simulink model "Main_simulation_gio"  (R2021b)
settings: Solver=FixedStepAuto  StartTime=0.0  StopTime=Time  FixedStep=0.1  RelTol=1e-13  AbsTol=1e-19
values from neighbouring files (symbols this model uses):
  a = 8.6251e06    (= 8625100)    [main_code.m]
  A_BN_0 = eye(3)    [main_code.m]
  A_rw = [1 0 0 1/sqrt(3);         0 1 0 1/sqrt(3) ... (first row only)    [main_code.m]
  A_rw_star = [5/6 -1/6 -1/6;              -1/6  5/6 -1/6 ... (first row only)    [main_code.m]
  c = 2.99792*10^8    (= 299792000)    [main_code.m]
  e = 0.1195    [main_code.m]
  G = [gn, gm, gvali, gsvi]    [main_code.m]
  H = [hn, hm, hvali, hsvi]    [main_code.m]
  i = 0.3815    [main_code.m]
  MB = [1; 0.3; 0.3; 0.3]    [main_code.m]
  mr = 1.2*1e-4    (= 0.00012)    [main_code.m]
  mu_P = G * Mt    (= 398527110340000)    [main_code.m]
  omega_0 = [w_0x; w_0y; w_0z]    [main_code.m]
  p_acc = 0.5    [main_code.m]
  rho_d_MB = 0.1    [main_code.m]
  rho_d_SP = 0.1    [main_code.m]
  rho_s_MB = 0.5    [main_code.m]
  rho_s_SP = 0.1    [main_code.m]
  sig_b = sig_b^2    [main_code.m]
  sig_n = 0.15*pi/180/3600/sqrt(t_sample)    [main_code.m]
  SP = [3; 0.3; 1; 0.1]    [main_code.m]
  T = 2*pi / n    [main_code.m]
  t_sample = 1    [main_code.m]
  theta_0 = 0    [main_code.m]
undefined symbols (not defined in the file or in its folder): magnitude, theta0
libraries: matrix_library x13, vrlib x7, simulink x3, simulink_extras x1
(part 1 of 5)
settings Model: SimulationMode=accelerator  Creator=adity  LastModifiedBy=adity
settings SolverCC: ZeroCrossControl=DisableAll

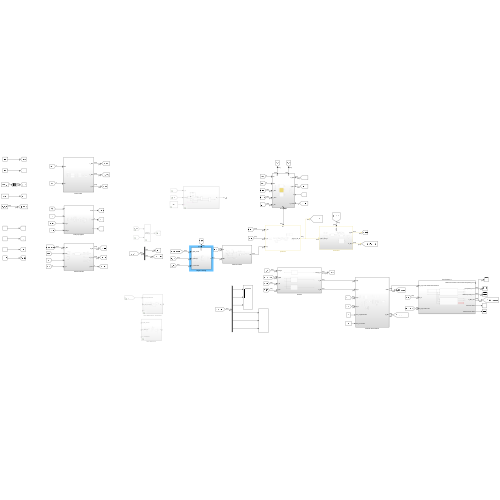
[thumbnail: Simulink's stored preview of the top-level diagram]
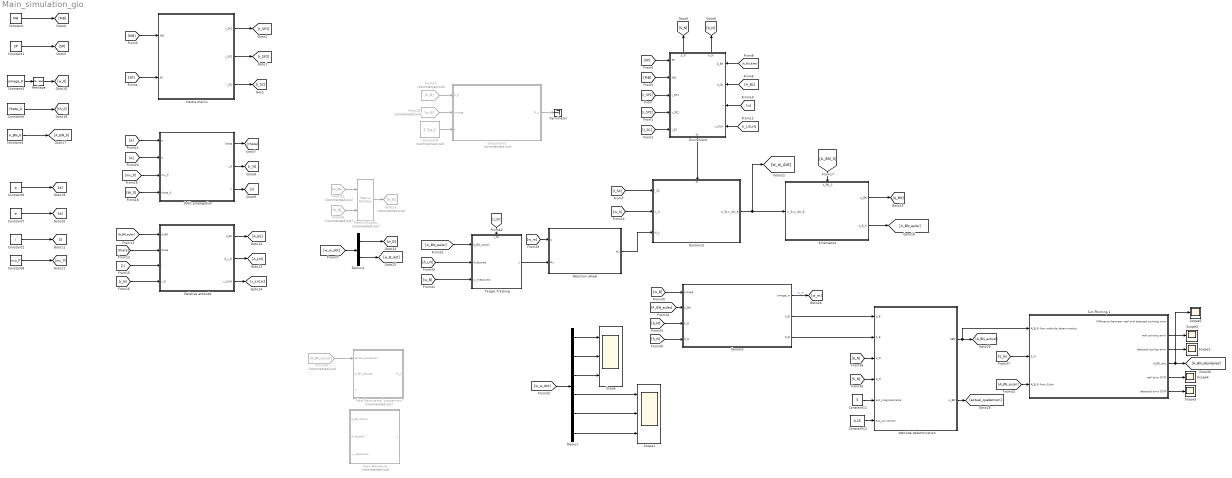
== system Main_simulation_gio ==
  Attitude determination : Subsystem
  Constant : Constant  Value=MB
  Constant1 : Constant  Value=SP
  Constant11 : Constant  Value=5
  Constant12 : Constant  Value=0.25
  Constant2 : Constant  Value=i
  Constant3 : Constant  Value=omega_0
  Constant4 : Constant  Value=A_BN_0
  Constant5 : Constant  Value=theta_0
  Constant6 : Constant  Value=a
  Constant7 : Constant  Value=e
  Constant8 : Constant  Value=mu_P
  Constant9 : Constant  Commented=on  Value=3.5e-2
  Demux : Demux  Outputs=6
  Demux1 : Demux  Outputs=2
  Dynamics : Subsystem
      settings: PortSchema="{\"entries\":[{\"content\":{\"sides\":[{\"content\":{\"connectorIds\":[\"In1\",\"In2\",\"In3\"]},\"type\":\"ConnectorPlacement.EquallySpacedRectSide\",\"uuid\":\"0fb0fd28-732a-45b7-951f-4b0b2306202c\"},{\"content\":{\"connectorIds\":[\"Out1\"],\"side\":\"RIGHT\"},\"type\":\"ConnectorPlacement.EquallySpacedRectSide\",\"uuid\":\"160a6d95-5e8b-4088-9ac4-372e2ef53b1e\"},{\"content\":{\"connectorIds\":[\"In4\"],\"side\":\"TOP\"},\"type\":\"ConnectorPlacement.EquallySpacedRectSide\",\"uuid\":\"bc0d773d-9b3c-40c2-804a-fc9efd6e220c\"}]},\"type\":\"ConnectorPlacement.EquallySpacedConnector\",\"uuid\":\"1f85a25c-c8d4-4d9d-9994-483d99135538\"}],\"packageUris\":[\"http://schema.mathworks.com/mf0/Connector/R2020b\"],\"version\":\"1.0\"}"
  Enviroment : Subsystem
      settings: PortSchema="{\"entries\":[{\"content\":{\"sides\":[{\"content\":{\"connectorIds\":[\"Out2\",\"Out3\"]},\"type\":\"ConnectorPlacement.EquallySpacedRectSide\",\"uuid\":\"77a65197-c5ef-4c05-af97-bd670bb59a1b\"},{\"content\":{\"connectorIds\":[\"Out1\"],\"side\":\"RIGHT\"},\"type\":\"ConnectorPlacement.EquallySpacedRectSide\",\"uuid\":\"f4905732-994b-44e8-915f-1f1165b6d340\"},{\"content\":{\"connectorIds\":[\"In1\",\"In2\",\"In3\",\"In4\",\"In5\"],\"side\":\"TOP\"},\"type\":\"ConnectorPlacement.EquallySpacedRectSide\",\"uuid\":\"dbb628bc-072b-4daa-a580-a056bf799753\"},{\"content\":{\"connectorIds\":[\"In6\",\"In7\",\"In8\",\"In9\"],\"side\":\"BOTTOM\"},\"type\":\"ConnectorPlacement.EquallySpacedRectSide\",\"uuid\":\"e6af6235-b92e-4098-9bbc-91b77f168ead\"}]},\"type\":\"ConnectorPlacement.EquallySpacedConnector\",\"uuid\":\"a4645f0d-8f51-4ba7-9ec5-d423e83ccc17\"}],\"packageUris\":[\"http://schema.mathworks.com/mf0/Connector/R2020b\"],\"version\":\"1.0\"}"
  From22 : From  Commented=on  GotoTag=A_BN
  From23 : From  Commented=on  GotoTag=b_B
  From26 : From  Commented=on  GotoTag=b_N
  From28 : From  Commented=on  GotoTag=w_B
  From38 : From  Commented=on  GotoTag=A_BN_actual
  Goto23 : Goto  Commented=on  GotoTag=b_B
  Inertia matrix : Subsystem
  Kinematics : Subsystem
      settings: PortSchema="{\"entries\":[{\"content\":{\"sides\":[{\"content\":{\"connectorIds\":[\"In1\"]},\"type\":\"ConnectorPlacement.EquallySpacedRectSide\",\"uuid\":\"b4580536-f47d-4a76-9d7a-ad9e45e6fd22\"},{\"content\":{\"connectorIds\":[\"Out1\",\"Out2\"],\"side\":\"RIGHT\"},\"type\":\"ConnectorPlacement.EquallySpacedRectSide\",\"uuid\":\"4273ed6e-d469-4a82-9e71-da4fb1c9f709\"},{\"content\":{\"connectorIds\":[\"In2\"],\"side\":\"TOP\"},\"type\":\"ConnectorPlacement.EquallySpacedRectSide\",\"uuid\":\"bac57a2b-a638-4d55-8f6f-550bb52319aa\"}]},\"type\":\"ConnectorPlacement.EquallySpacedConnector\",\"uuid\":\"29527554-7b77-4957-9d93-347c44cffae5\"}],\"packageUris\":[\"http://schema.mathworks.com/mf0/Connector/R2020b\"],\"version\":\"1.0\"}"
  Matrix Multiply : Product  Commented=on  Multiplication=Matrix(*)
  Orbit propagation : Subsystem
  Reaction wheel : Subsystem
  Relative attitude : Subsystem
  Reshape : Reshape  OutputDimensionality=Column vector (2-D)
  Scope : Scope  NumInputPorts=3
  Scope1 : Scope  NumInputPorts=3
  Scope{2..6} (5 alike) : Scope
  Sensors : Subsystem
  Slew Manoevre : Subsystem  Commented=on
  "Slew Manouevre \"quaternion\"" : Subsystem  Commented=on
  Subsystem1 : Subsystem  Commented=on
  Sun Pointing 1 : Subsystem
  Target Tracking : Subsystem
      settings: PortSchema="{\"entries\":[{\"content\":{\"sides\":[{\"content\":{\"connectorIds\":[\"In1\",\"In2\",\"In3\"]},\"type\":\"ConnectorPlacement.EquallySpacedRectSide\",\"uuid\":\"1538af5c-7ca3-4c69-907f-3af05bd2e46a\"},{\"content\":{\"connectorIds\":[\"Out1\"],\"side\":\"RIGHT\"},\"type\":\"ConnectorPlacement.EquallySpacedRectSide\",\"uuid\":\"fe4d23c6-7042-48db-bda4-c7db1868d73a\"},{\"content\":{\"connectorIds\":[\"In4\"],\"side\":\"TOP\"},\"type\":\"ConnectorPlacement.EquallySpacedRectSide\",\"uuid\":\"8091eb5d-cc3c-4ce8-99cb-f347939312a6\"}]},\"type\":\"ConnectorPlacement.EquallySpacedConnector\",\"uuid\":\"01b1afd0-a44e-4fda-a912-00799ef3cdac\"}],\"packageUris\":[\"http://schema.mathworks.com/mf0/Connector/R2020b\"],\"version\":\"1.0\"}"
  Terminator : Terminator
  wires:
  Inertia matrix/3(I_SC) -> [I_SC]
  Inertia matrix/2(r_SP2) -> [r_SP2]
  Inertia matrix/1(r_SP1) -> [r_SP1]
  [r_SP1] -> Enviroment/3(r_SP1)
  [r_SP2] -> Enviroment/4(r_SP2)
  [I_SC] -> Enviroment/5(I_SC)
  Constant/1 -> [MB]
  Constant1/1 -> [SP]
  [MB] -> Inertia matrix/1(MB)
  [SP] -> Inertia matrix/2(SP)
  [MB] -> Enviroment/2(MB)
  [SP] -> Enviroment/1(SP)
  Enviroment/1(M) -> Dynamics/4(M)
  [I_SC] -> Dynamics/1(I_SC)
  Enviroment/2(S_N) -> [S_N]
  Enviroment/3(b_N) -> [b_N]
  [A_BN_euler] -> Enviroment/6(A_BN)
  [A_BL] -> Enviroment/7(A_BL)
  [n] -> Enviroment/8(n)
  [r_LVLH] -> Enviroment/9(r_LVLH)
  Orbit propagation/1(theta) -> [theta]
  Orbit propagation/2(r_N) -> [r_N]
  Orbit propagation/3(n) -> [n]
  [theta] -> Relative attitude/2(theta)
  [A_BN_euler] -> Relative attitude/1(A_BN)
  [w_0] -> Dynamics/2(w_0)
  Constant2/1 -> [i]
  [i] -> Relative attitude/3(i)
  Relative attitude/1(A_BL) -> [A_BL]
  Relative attitude/2(A_L_N) -> [A_LN]
  Dynamics/1(w_B,w_dot_B) -> [w_w_dot], Kinematics/1(w_B,w_dot_B)
  [r_N] -> Relative attitude/4(r_N)
  Relative attitude/3(r_LVLH) -> [r_LVLH]
  Kinematics/1(q_BN) -> [q_BN]
  Kinematics/2(A_B_N) -> [A_BN_euler]
  [A_BN_0] -> Kinematics/2(A_BN_0)
  Constant4/1 -> [A_BN_0]
  Constant5/1 -> [th_0]
  [th_0] -> Orbit propagation/4(theta_0)
  Constant6/1 -> [a]
  Constant7/1 -> [e]
  Constant8/1 -> [mu_P]
  [mu_P] -> Orbit propagation/3(mu_P)
  [e] -> Orbit propagation/2(e)
  [a] -> Orbit propagation/1(a)
  Demux/1 -> Scope/1
  Demux/2 -> Scope/2
  Demux/3 -> Scope/3
  Demux/4 -> Scope1/1
  Demux/5 -> Scope1/2
  Demux/6 -> Scope1/3
  [w_w_dot] -> Demux/1
  From22/1 -> Matrix Multiply/1
  From26/1 -> Matrix Multiply/2
  Matrix Multiply/1 -> Goto23/1
  From23/1 -> Subsystem1/1(b_b)
  [w_w_dot] -> Demux1/1
  Demux1/1 -> [w_B]
  Demux1/2 -> [w_B_dot]
  Constant9/1 -> Subsystem1/3(K)
  From28/1 -> Subsystem1/2(omega)
  Constant3/1 -> Reshape/1
  Reshape/1 -> [w_0]
  Target Tracking/1(u) -> Reaction wheel/2(Mc)
  Reaction wheel/1(Mr) -> Dynamics/3(M_c)
  From38/1 -> "Slew Manouevre \"quaternion\""/1(actual quaternion)
  [w_m] -> Reaction wheel/1(w)
  [A_LN] -> Target Tracking/2(A_desired)
  [w_B] -> Target Tracking/3(w_measured)
  Subsystem1/1(M_c) -> Terminator/1
  [w_B] -> Sensors/1(omega)
  [A_BN_euler] -> Sensors/2(A_BN)
  [b_N] -> Sensors/3(b_N)
  [S_N] -> Sensors/4(S_N)
  Sensors/1(omega_m) -> [w_m]  "w_m"
  Sensors/2(b_B) -> Attitude determination/1(b_B)
  Sensors/3(S_B) -> Attitude determination/2(S_B)
  Constant12/1 -> Attitude determination/6(acc_sun sensor)
  Constant11/1 -> Attitude determination/5(acc_magnetometre)
  [S_N] -> Attitude determination/4(S_N)
  [b_N] -> Attitude determination/3(b_N)
  Sun Pointing 1/4(A_BN_des) -> Scope6/1, [A_BN_desidered]
  [S_N] -> Sun Pointing 1/2(S_N)
  [A_BN_euler] -> Sun Pointing 1/3(A_B_N from Euler)
  Attitude determination/1(ABN) -> Sun Pointing 1/1(A_B_N from attitude determination), [A_BN_actual]
  Sun Pointing 1/3(detected pointig error) -> Scope2/1
  Sun Pointing 1/2(real pointing error) -> Scope3/1
  Sun Pointing 1/5(real error DCM) -> Scope4/1
  Sun Pointing 1/6(detected error DCM) -> Scope5/1
  Attitude determination/2(q_BN) -> [actual_quaternion]
  [A_BN_euler] -> Target Tracking/1(A_BN_actual)
  [I_SC] -> Target Tracking/4(I_SC)

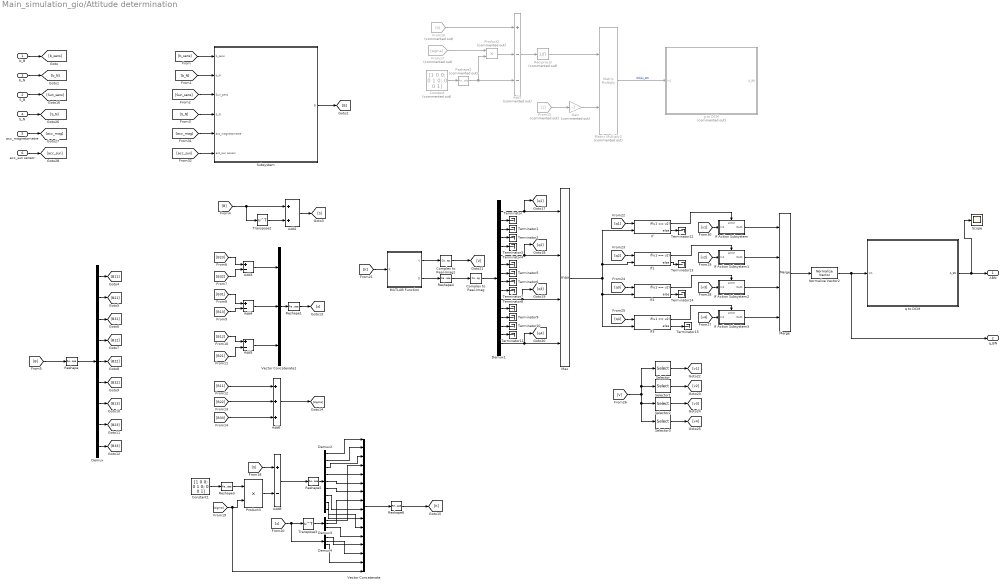
== system Main_simulation_gio/Attitude determination ==
  b_B : Inport
  S_B : Inport  Port=2
  b_N : Inport  Port=3
  S_N : Inport  Port=4
  acc_magnetometre : Inport  Port=5
  acc_sun sensor : Inport  Port=6
  Add2 : Sum
  Add{3..5,8} (4 alike) : Sum  Inputs=+-
  Add6 : Sum  Inputs=+++
  Add7 : Sum  Commented=on  Inputs=+--
  Complex to Real-Imag : ComplexToRealImag  Output=Real
  Complex to Real-Imag1 : ComplexToRealImag  Output=Real
  Constant : Constant  Commented=on  Value=[1 0 0; 0 1 0; 0 0 1]  VectorParams1D=off
  Constant1 : Constant  Value=[1 0 0; 0 1 0; 0 0 1]  VectorParams1D=off
  Demux : Demux  Outputs=9
  Demux1 : Demux  Outputs=16
  Demux2 : Demux  Outputs=9
  Demux3 : Demux  Outputs=3
  Demux4 : Demux  Outputs=3
  From15 : From  Commented=on  GotoTag=z
  From16 : From  Commented=on  GotoTag=S
  From17 : From  Commented=on  GotoTag=sigma
  Gain : Gain  Commented=on  Gain=-1
  If{,1..3} (4 alike) : If  NumInputs=2  IfExpression=u1 == u2
  If Action Subsystem : Subsystem  TreatAsAtomicUnit=on
  If Action Subsystem1 : Subsystem  TreatAsAtomicUnit=on
  If Action Subsystem2 : Subsystem  TreatAsAtomicUnit=on
  If Action Subsystem3 : Subsystem  TreatAsAtomicUnit=on
  MATLAB Function : MATLAB Function  TreatAsAtomicUnit=on
  Matrix Multiply2 : Product  Commented=on  Multiplication=Matrix(*)
  Max : MinMax  Function=max  Inputs=4
  Merge : Merge  Inputs=4
  Normalize Vector2 : vrlib/Utilities/Normalize Vector  maxzero=0
  Product2 : Product  Commented=on
  Product3 : Product
  Reciprocal : Product  Commented=on  Inputs=/
  Reshape{,1,4..5} (4 alike) : Reshape  OutputDimensionality=Column vector (2-D)
  Reshape2 : Reshape  Commented=on  OutputDimensionality=Customize  OutputDimensions=[3,3]
  Reshape3 : Reshape  OutputDimensionality=Customize  OutputDimensions=[3,3]
  Reshape6 : Reshape  OutputDimensionality=Customize  OutputDimensions=[4,4]
  Scope : Scope
  Selector : Selector  NumberOfDimensions=2  InputPortWidth=3  IndexOptions=Index vector (dialog),Index vector (dialog)  Indices=[1 2 3 4],1  OutputSizes=1,1
  Selector1 : Selector  NumberOfDimensions=2  InputPortWidth=3  IndexOptions=Index vector (dialog),Index vector (dialog)  Indices=[1 2 3 4],2  OutputSizes=1,1
  Selector2 : Selector  NumberOfDimensions=2  InputPortWidth=3  IndexOptions=Index vector (dialog),Index vector (dialog)  Indices=[1 2 3 4],3  OutputSizes=1,1
  Selector3 : Selector  NumberOfDimensions=2  InputPortWidth=3  IndexOptions=Index vector (dialog),Index vector (dialog)  Indices=[1 2 3 4],4  OutputSizes=1,1
  Subsystem : Subsystem
  Terminator{,1..15} (16 alike) : Terminator
  Transpose2 : Math  Operator=transpose  SaturateOnIntegerOverflow=on
  Transpose3 : Math  Operator=transpose  SaturateOnIntegerOverflow=on
  Vector Concatenate : Concatenate  NumInputs=16
  Vector Concatenate1 : Concatenate  NumInputs=3
  g to DCM : Subsystem  Commented=on
  q to DCM : Subsystem
  ABN : Outport
  q_BN : Outport  Port=2
  wires:
  [B] -> Transpose2/1, Add2/1
  Transpose2/1 -> Add2/2
  Add2/1 -> [S]
  [B] -> Reshape/1
  Reshape/1 -> Demux/1
  Demux/1 -> [B11]
  Demux/2 -> [B21]
  Demux/3 -> [B31]
  Demux/4 -> [B12]
  Demux/5 -> [B22]
  Demux/6 -> [B32]
  Demux/7 -> [B13]
  Demux/8 -> [B23]
  Demux/9 -> [B33]
  [B23] -> Add3/1
  [B32] -> Add3/2
  [B31] -> Add4/1
  [B13] -> Add4/2
  [B12] -> Add5/1
  [B21] -> Add5/2
  Add3/1 -> Vector Concatenate1/1
  Add4/1 -> Vector Concatenate1/2
  Add5/1 -> Vector Concatenate1/3
  Vector Concatenate1/1 -> Reshape1/1
  Reshape1/1 -> [z]
  [B11] -> Add6/1
  [B22] -> Add6/2
  [B33] -> Add6/3
  Add6/1 -> [sigma]
  From15/1 -> Gain/1
  Constant/1 -> Reshape2/1
  From17/1 -> Product2/1
  Reshape2/1 -> Add7/3, Product2/2
  From16/1 -> Add7/1
  Product2/1 -> Add7/2
  Add7/1 -> Reciprocal/1
  Reciprocal/1 -> Matrix Multiply2/1
  Gain/1 -> Matrix Multiply2/2
  Matrix Multiply2/1 -> g to DCM/1(In1)  "Gibbs_BN"
  Constant1/1 -> Reshape3/1
  Reshape3/1 -> Product3/1
  [sigma] -> Vector Concatenate/16, Product3/2
  Product3/1 -> Add8/2
  [S] -> Add8/1
  Add8/1 -> Reshape5/1
  MATLAB Function/2(D) -> Reshape4/1
  Demux1/2 -> Terminator/1
  Demux1/3 -> Terminator1/1
  Demux1/4 -> Terminator2/1
  Demux1/5 -> Terminator3/1
  Demux1/6 -> [q2], Max/2
  Demux1/7 -> Terminator4/1
  Demux1/8 -> Terminator5/1
  Demux1/9 -> Terminator6/1
  Demux1/10 -> Terminator7/1
  Demux1/11 -> [q3], Max/3
  Demux1/16 -> [q4], Max/4
  Demux1/12 -> Terminator8/1
  Demux1/13 -> Terminator9/1
  Demux1/14 -> Terminator10/1
  Demux1/15 -> Terminator11/1
  Reshape4/1 -> Complex to Real-Imag/1
  Max/1 -> If3/2, If2/2, If1/2, If/2
  Demux1/1 -> [q1], Max/1
  [q1] -> If/1
  [q2] -> If1/1
  [q4] -> If3/1
  [q3] -> If2/1
  MATLAB Function/1(V) -> Complex to Real-Imag1/1
  Selector1/1 -> [v2]
  Selector3/1 -> [v4]
  Selector2/1 -> [v3]
  Selector/1 -> [v1]
  [V] -> Selector/1, Selector1/1, Selector3/1, Selector2/1
  If/1 -> If Action Subsystem/Action
  If/2 -> Terminator12/1
  If1/2 -> Terminator13/1
  If2/2 -> Terminator14/1
  If3/2 -> Terminator15/1
  If Action Subsystem/1(Out1) -> Merge/1
  If1/1 -> If Action Subsystem1/Action
  If2/1 -> If Action Subsystem2/Action
  If3/1 -> If Action Subsystem3/Action
  If Action Subsystem3/1(Out1) -> Merge/4
  If Action Subsystem2/1(Out1) -> Merge/3
  If Action Subsystem1/1(Out1) -> Merge/2
  [v4] -> If Action Subsystem3/1(In1)
  [v1] -> If Action Subsystem/1(In1)
  [v2] -> If Action Subsystem1/1(In1)
  [v3] -> If Action Subsystem2/1(In1)
  q to DCM/1(A_BN) -> Scope/1, ABN/1
  Merge/1 -> Normalize Vector2/1
  Reshape5/1 -> Demux2/1
  Demux2/1 -> Vector Concatenate/1
  Demux2/2 -> Vector Concatenate/2
  Demux2/3 -> Vector Concatenate/3
  [z] -> Demux4/1, Transpose3/1
  Transpose3/1 -> Demux3/1
  Demux3/1 -> Vector Concatenate/4
  Demux2/4 -> Vector Concatenate/5
  Demux2/5 -> Vector Concatenate/6
  Demux2/6 -> Vector Concatenate/7
  Demux3/2 -> Vector Concatenate/8
  Demux2/7 -> Vector Concatenate/9
  Demux2/8 -> Vector Concatenate/10
  Demux2/9 -> Vector Concatenate/11
  Demux3/3 -> Vector Concatenate/12
  Demux4/2 -> Vector Concatenate/14
  Demux4/1 -> Vector Concatenate/13
  Demux4/3 -> Vector Concatenate/15
  Vector Concatenate/1 -> Reshape6/1
  Reshape6/1 -> [K]
  Complex to Real-Imag/1 -> Demux1/1
  Normalize Vector2/1 -> q_BN/1, q to DCM/1(In1)
  Complex to Real-Imag1/1 -> [V]
  [K] -> MATLAB Function/1(K)
  Subsystem/1(B) -> [B]
  b_B/1 -> [b_sens]
  b_N/1 -> [b_N]
  S_B/1 -> [Sun_sens]
  S_N/1 -> [S_N]
  acc_magnetometre/1 -> [acc_mag]
  acc_sun sensor/1 -> [acc_sun]
  [b_sens] -> Subsystem/1(b_sens)
  [b_N] -> Subsystem/2(b_N)
  [Sun_sens] -> Subsystem/3(Sun_sens)
  [S_N] -> Subsystem/4(S_N)
  [acc_mag] -> Subsystem/5(acc_magnetometre)
  [acc_sun] -> Subsystem/6(acc_sun sensor)

== system Main_simulation_gio/Dynamics ==
  I_SC : Inport
  w_0 : Inport  Port=2
  M_c : Inport  Port=3
  M : Inport  Port=4
  Add : Sum
  Cross Product : vrlib/Utilities/Cross Product
  Demux : Demux  Outputs=3
  Gain5 : Gain  Gain=-1
  Integrator4 : Integrator  InitialConditionSource=external  InitialCondition=omega_0
  Mux : Mux  Inputs=2
  Product6 : Product  Multiplication=Matrix(*)
  Product7 : Product  Multiplication=Matrix(*)
  Reciprocal : Product  Inputs=/  Multiplication=Matrix(*)
  Scope : Scope  NumInputPorts=3
  Scope1 : Scope
  Sum2 : Sum
  w_B,w_dot_B : Outport
  wires:
  Sum2/1 -> Product7/2
  Product6/1 -> Cross Product/2
  Product7/1 -> [w_dot_B], Integrator4/1
  Cross Product/1 -> Gain5/1
  Gain5/1 -> Sum2/1
  Integrator4/1 -> [w_B], Demux/1, Cross Product/1, Product6/2
  I_SC/1 -> [I_SC]
  [I_SC] -> Product6/1
  [I_SC] -> Reciprocal/1
  Reciprocal/1 -> Product7/1
  w_0/1 -> [w_0]
  [w_0] -> Integrator4/2
  Demux/2 -> Scope/2  "om_y"
  Demux/1 -> Scope/1  "om_x"
  Demux/3 -> Scope/3  "om_z"
  Add/1 -> Sum2/2
  M_c/1 -> Add/2
  Mux/1 -> w_B,w_dot_B/1
  [w_B] -> Mux/1
  [w_dot_B] -> Mux/2
  M/1 -> Add/1, Scope1/1

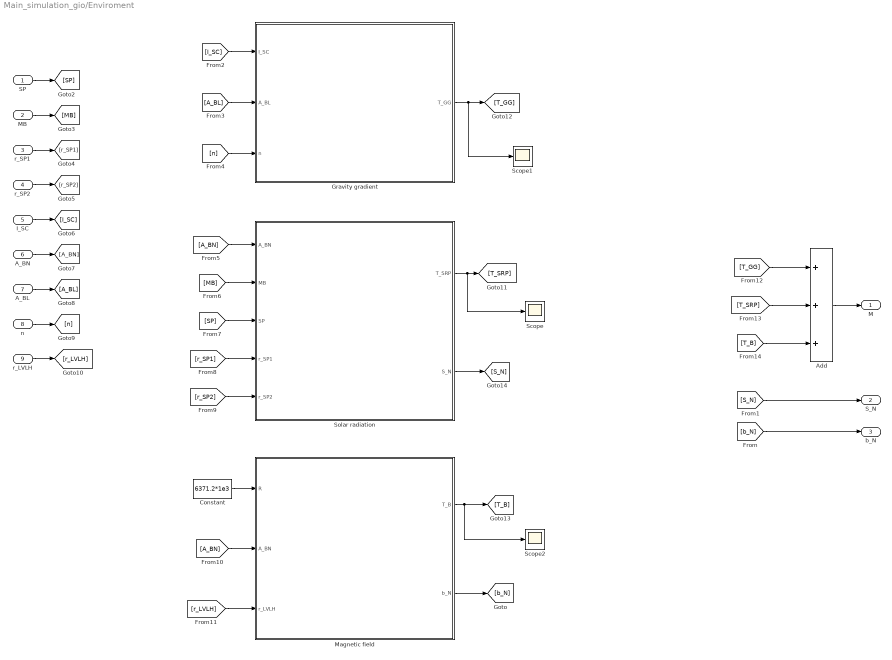
== system Main_simulation_gio/Enviroment ==
  SP : Inport
  MB : Inport  Port=2
  r_SP1 : Inport  Port=3
  r_SP2 : Inport  Port=4
  I_SC : Inport  Port=5
  A_BN : Inport  Port=6
  A_BL : Inport  Port=7
  n : Inport  Port=8
  r_LVLH : Inport  Port=9
  Add : Sum  Inputs=+++
  Constant : Constant  Value=6371.2*1e3
  Gravity gradient : Subsystem
  Magnetic field : Subsystem
  Scope : Scope
  Scope1 : Scope
  Scope2 : Scope
  Solar radiation : Subsystem
  M : Outport
  S_N : Outport  Port=2
  b_N : Outport  Port=3
  wires:
  Add/1 -> M/1
  Constant/1 -> Magnetic field/1(R)
  [b_N] -> b_N/1
  [S_N] -> S_N/1
  SP/1 -> [SP]
  MB/1 -> [MB]
  r_SP1/1 -> [r_SP1]
  r_SP2/1 -> [r_SP2]
  I_SC/1 -> [I_SC]
  A_BN/1 -> [A_BN]
  A_BL/1 -> [A_BL]
  n/1 -> [n]
  r_LVLH/1 -> [r_LVLH]
  Magnetic field/2(b_N) -> [b_N]
  Solar radiation/1(T_SRP) -> Scope/1, [T_SRP]
  Gravity gradient/1(T_GG) -> Scope1/1, [T_GG]
  Magnetic field/1(T_B) -> Scope2/1, [T_B]
  [I_SC] -> Gravity gradient/1(I_SC)
  [A_BL] -> Gravity gradient/2(A_BL)
  [n] -> Gravity gradient/3(n)
  [A_BN] -> Solar radiation/1(A_BN)
  [MB] -> Solar radiation/2(MB)
  [SP] -> Solar radiation/3(SP)
  [r_SP1] -> Solar radiation/4(r_SP1)
  [r_SP2] -> Solar radiation/5(r_SP2)
  [A_BN] -> Magnetic field/2(A_BN)
  [r_LVLH] -> Magnetic field/3(r_LVLH)
  Solar radiation/2(S_N) -> [S_N]
  [T_GG] -> Add/1
  [T_SRP] -> Add/2
  [T_B] -> Add/3

== system Main_simulation_gio/Inertia matrix ==
  note: I_SP is for 2 solar panels
  note: a lato corto, b lato lungo h spessore
      | lato lungo asse x solar panel
      | lato corto asse z solar panel
      | lato lungo asse y main body
      | lato corto asse x main body
      | spessore asse z main body
  MB : Inport
  SP : Inport  Port=2
  Complex to Real-Imag : ComplexToRealImag  Output=Real
  Constant : Constant  Value=[19.5 0 0; 0 19 0; 0 0 12.6]  VectorParams1D=off
  Demux : Demux
  Demux1 : Demux
  MATLAB Function : MATLAB Function  TreatAsAtomicUnit=on
  Main body : Subsystem
  Reshape : Reshape  OutputDimensionality=Customize  OutputDimensions=[3,3]
  Solar panel : Subsystem
  Sum : Sum
  Terminator : Terminator
  Terminator1 : Terminator
  Transport theorem : Subsystem
  r_SP : Subsystem
  r_SP1 : Outport
  r_SP2 : Outport  Port=2
  I_SC : Outport  Port=3
  wires:
  MB/1 -> Demux1/1
  Demux/1 -> [m_SP]
  Transport theorem/1(I_SP_B) -> Sum/1
  [r_SP1] -> Transport theorem/2(r_SP)
  Main body/1(I_MB) -> Sum/2
  [m_SP] -> Transport theorem/3(m_SP)
  r_SP/1(r_SP1) -> [r_SP1]
  [r_SP1] -> r_SP1/1
  [r_SP2] -> r_SP2/1
  r_SP/2(r_SP2) -> [r_SP2]
  Demux/2 -> [a_SP]
  Demux/3 -> [b_SP]
  Demux/4 -> [h_SP]
  [a_SP] -> Solar panel/2(a_SP)
  [b_SP] -> Solar panel/3(b_SP)
  [m_SP] -> Solar panel/1(m_SP)
  [h_SP] -> Solar panel/4(h_SP)
  [b_SP] -> r_SP/1(b_SP)
  Demux1/4 -> [h_MB]
  Demux1/3 -> [b_MB]
  Demux1/2 -> [a_MB]
  Demux1/1 -> [m_MB]
  [m_MB] -> Main body/1(m_MB)
  [a_MB] -> Main body/2(a_MB)
  [b_MB] -> Main body/3(b_MB)
  [h_MB] -> Main body/4(h_MB)
  [a_MB] -> r_SP/2(a_MB)
  Solar panel/1(I_SP) -> [I_SP]
  SP/1 -> Demux/1
  [I_SC] -> I_SC/1
  [I_SP] -> Transport theorem/1(I_SP)
  Sum/1 -> MATLAB Function/1(u)
  MATLAB Function/1(V) -> Terminator/1
  MATLAB Function/2(D) -> Complex to Real-Imag/1
  Complex to Real-Imag/1 -> Terminator1/1
  Constant/1 -> Reshape/1
  Reshape/1 -> [I_SC]

== system Main_simulation_gio/Kinematics ==
  w_B,w_dot_B : Inport
  A_BN_0 : Inport  Port=2
  DCM to quaternion : Subsystem
  Demux : Demux  Outputs=2
  Gain : Gain  Gain=1/2
  Integrator : Integrator  InitialConditionSource=external  InitialCondition=[0; 0; 0; 1]
  Matrix Multiply : Product  Multiplication=Matrix(*)
  Normalisation : Subsystem
  Reshape : Reshape  OutputDimensionality=Column vector (2-D)
  Subsystem : Subsystem
  Terminator : Terminator
  q to DCM : Subsystem
  q_BN : Outport
  A_B_N : Outport  Port=2
  wires:
  w_B,w_dot_B/1 -> Demux/1
  Demux/1 -> [w_B]
  Demux/2 -> Terminator/1
  A_BN_0/1 -> [A_BN_0]
  [q_0] -> Integrator/2
  [w_B] -> Subsystem/1(w_B)
  DCM to quaternion/1(q) -> [q_0]
  Subsystem/1(OMEGA) -> [OMEGA]
  Reshape/1 -> Normalisation/1(In1)
  Integrator/1 -> Reshape/1  "q(t)"
  [OMEGA] -> Gain/1
  Gain/1 -> Matrix Multiply/1
  Normalisation/1(Out1) -> Matrix Multiply/2, [q_BN]  "q(t)"
  Matrix Multiply/1 -> Integrator/1  "dq/dt"
  [A_BN_0] -> DCM to quaternion/1(DCM)
  [q_BN] -> q_BN/1
  [A_BN] -> A_B_N/1
  q to DCM/1(A_BN) -> [A_BN]
  [q_BN] -> q to DCM/1(q_BN)

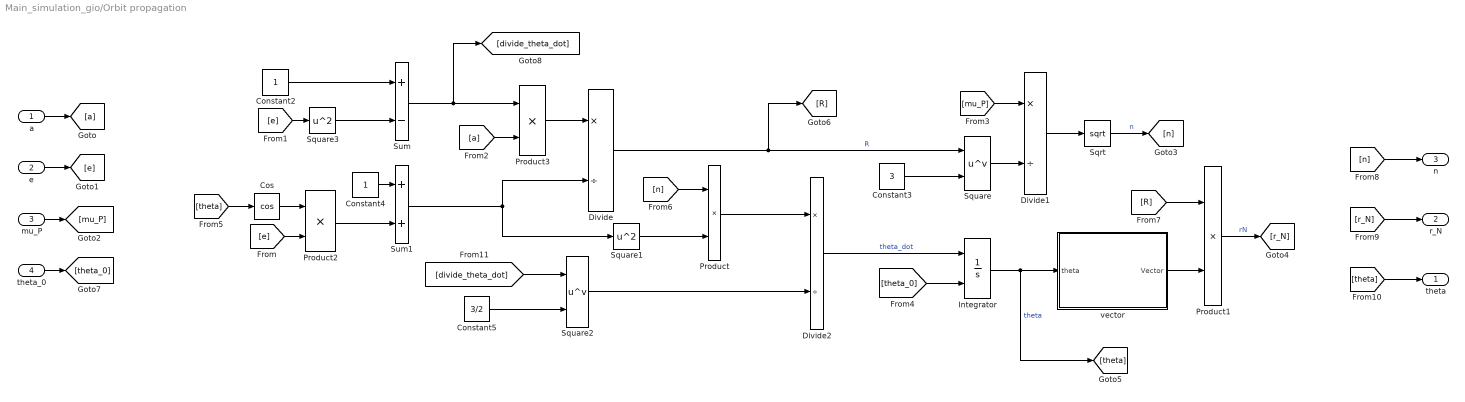
== system Main_simulation_gio/Orbit propagation ==
  a : Inport
  e : Inport  Port=2
  mu_P : Inport  Port=3
  theta_0 : Inport  Port=4
  Constant2 : Constant
  Constant3 : Constant  Value=3
  Constant4 : Constant
  Constant5 : Constant  Value=3/2
  Cos : Trigonometry  Operator=cos
  Divide : Product  Inputs=*/
  Divide1 : Product  Inputs=*/
  Divide2 : Product  Inputs=*/
  Integrator : Integrator  InitialConditionSource=external  InitialCondition=theta0
  Product{,1..3} (4 alike) : Product
  Sqrt : Sqrt  SaturateOnIntegerOverflow=on
  Square : Math  Operator=pow  SaturateOnIntegerOverflow=on
  Square1 : Math  Operator=square  SaturateOnIntegerOverflow=on
  Square2 : Math  Operator=pow  SaturateOnIntegerOverflow=on
  Square3 : Math  Operator=square  SaturateOnIntegerOverflow=on
  Sum : Sum  Inputs=+-
  Sum1 : Sum
  vector : Subsystem
  theta : Outport
  r_N : Outport  Port=2
  n : Outport  Port=3
  wires:
  Constant2/1 -> Sum/1
  Square3/1 -> Sum/2
  Sum/1 -> [divide_theta_dot], Product3/1
  Product3/1 -> Divide/1
  Constant4/1 -> Sum1/1
  Sum1/1 -> Square1/1, Divide/2
  Product2/1 -> Sum1/2
  Cos/1 -> Product2/1
  Integrator/1 -> [theta], vector/1(theta)  "theta"
  Divide1/1 -> Sqrt/1
  [mu_P] -> Divide1/1
  Square/1 -> Divide1/2
  Divide/1 -> [R], Square/1  "R"
  Constant3/1 -> Square/2
  Sqrt/1 -> [n]  "n"
  Square1/1 -> Product/2
  Constant5/1 -> Square2/2
  Product/1 -> Divide2/1
  Divide2/1 -> Integrator/1  "theta_dot"
  vector/1(Vector) -> Product1/2
  Square2/1 -> Divide2/2
  a/1 -> [a]
  e/1 -> [e]
  mu_P/1 -> [mu_P]
  [e] -> Product2/2
  [e] -> Square3/1
  [a] -> Product3/2
  [theta_0] -> Integrator/2
  Product1/1 -> [r_N]  "rN"
  [theta] -> Cos/1
  [n] -> Product/1
  [R] -> Product1/1
  [n] -> n/1
  [r_N] -> r_N/1
  [theta] -> theta/1
  theta_0/1 -> [theta_0]
  [divide_theta_dot] -> Square2/1

== system Main_simulation_gio/Reaction wheel ==
  w : Inport
  Mc : Inport  Port=2
  A : Constant  Value=A_rw
  A_star : Constant  Value=A_rw_star
  Add : Sum  Inputs=--
  Constant : Constant  Value=[0 0 0 0]
  Cross Product : matrix_library/Cross Product
      settings: SourceProductBaseCode=SL
  Cross Product1 : matrix_library/Cross Product
      settings: SourceProductBaseCode=SL
  Gain : Gain  Gain=-1
  Integrator : Integrator  InitialConditionSource=external
  Matrix Multiply{,1..3} (4 alike) : Product  Multiplication=Matrix(*)
  Reshape : Reshape  OutputDimensionality=Column vector (2-D)
  Reshape1 : Reshape  OutputDimensionality=Column vector (2-D)
  Sum : Sum  Inputs=|++
  Mr : Outport
  wires:
  Integrator/1 -> [h_r], Matrix Multiply/2
  A/1 -> [A_rw], Matrix Multiply/1
  w/1 -> [omega], Cross Product/1
  Matrix Multiply/1 -> Cross Product/2
  Cross Product/1 -> Sum/1
  Mc/1 -> Reshape1/1
  Sum/1 -> Matrix Multiply1/2
  A_star/1 -> Gain/1
  Gain/1 -> Matrix Multiply1/1
  Matrix Multiply1/1 -> Integrator/1, Matrix Multiply2/2
  Constant/1 -> Reshape/1
  Reshape/1 -> Integrator/2
  Reshape1/1 -> Sum/2
  [A_rw] -> Matrix Multiply2/1
  Matrix Multiply2/1 -> Add/1
  Add/1 -> Mr/1
  [omega] -> Cross Product1/1
  Matrix Multiply3/1 -> Cross Product1/2
  [A_rw] -> Matrix Multiply3/1
  [h_r] -> Matrix Multiply3/2
  Cross Product1/1 -> Add/2

== system Main_simulation_gio/Relative attitude ==
  A_BN : Inport
  theta : Inport  Port=2
  i : Inport  Port=3
  r_N : Inport  Port=4
  A_LN : Subsystem
  MatrixMultiply : Product  Multiplication=Matrix(*)
  MatrixMultiply1 : Product  Multiplication=Matrix(*)
  Transpose : Math  Operator=transpose  SaturateOnIntegerOverflow=on
  A_BL : Outport
  A_L_N : Outport  Port=2
  r_LVLH : Outport  Port=3
  wires:
  Transpose/1 -> MatrixMultiply/2
  MatrixMultiply/1 -> A_BL/1  "A_BL"
  theta/1 -> [theta]
  A_BN/1 -> [A_BN]
  [theta] -> A_LN/1(theta)
  A_LN/1(A_L_N) -> [A_LN]
  [i] -> A_LN/2(i)
  i/1 -> [i]
  [A_BN] -> MatrixMultiply/1
  [A_LN] -> Transpose/1
  [A_LN] -> A_L_N/1
  MatrixMultiply1/1 -> r_LVLH/1  "A_BL"
  [A_LN] -> MatrixMultiply1/1
  r_N/1 -> [r_N]
  [r_N] -> MatrixMultiply1/2

== system Main_simulation_gio/Sensors ==
  omega : Inport
  A_BN : Inport  Port=2
  b_N : Inport  Port=3
  S_N : Inport  Port=4
  Gyroscopes : Subsystem
  Magnetometer1 : Subsystem
  Sun sensor : Subsystem
  omega_m : Outport
  b_B : Outport  Port=2
  S_B : Outport  Port=3
  wires:
  omega/1 -> Gyroscopes/1(omega)
  Gyroscopes/1(omega_m) -> omega_m/1
  b_N/1 -> Magnetometer1/2(b_N)
  Magnetometer1/1(b_B) -> b_B/1
  Sun sensor/1(S_B) -> S_B/1
  A_BN/1 -> Sun sensor/2(A_BN), Magnetometer1/1(A_BN)
  S_N/1 -> Sun sensor/1(S_N)

== system Main_simulation_gio/Slew Manoevre ==
  A_BN_actual : Inport
  A_desired : Inport  Port=2
  w_measured : Inport  Port=3
  Demux : Demux  Outputs=3
  Gain : Gain  Gain=-1
  Gain1 : Gain  Gain=-1
  Matrix Multiply : Product  Multiplication=Matrix(*)
  Mux : Mux  Inputs=3
  Product : Product
  Product1 : Product
  Reshape : Reshape  OutputDimensionality=Customize  OutputDimensions=[3,1]
  Reshape1 : Reshape  OutputDimensionality=Column vector (2-D)
  Reshape2 : Reshape  OutputDimensionality=Column vector (2-D)
  Scope{,1..3} (4 alike) : Scope
  Selector : Selector  NumberOfDimensions=2  InputPortWidth=3  IndexOptions=Index vector (dialog),Index vector (dialog)  Indices=2,1  OutputSizes=1,1
  Selector1 : Selector  NumberOfDimensions=2  InputPortWidth=3  IndexOptions=Index vector (dialog),Index vector (dialog)  Indices=3,1  OutputSizes=1,1
  Selector2 : Selector  NumberOfDimensions=2  InputPortWidth=3  IndexOptions=Index vector (dialog),Index vector (dialog)  Indices=3,2  OutputSizes=1,1
  Sum : Sum  Inputs=|+|-|
  Sum1 : Sum  Inputs=|+|+|
  Terminator : Terminator
  Terminator1 : Terminator
  To Workspace : ToWorkspace  VariableName=error  SaveFormat=Timeseries  SampleTime=-1
  To Workspace1 : ToWorkspace  VariableName=omega  SaveFormat=Timeseries  SampleTime=-1
  Transpose : Math  Operator=transpose  SaturateOnIntegerOverflow=on
  Transpose1 : Math  Operator=transpose  SaturateOnIntegerOverflow=on
  k1 : Constant  Value=9.99e-2
  k2 : Constant  Value=1.25e-3
  u : Outport
  wires:
  Mux/1 -> Reshape/1, Demux/1, Scope/1
  w_measured/1 -> To Workspace1/1, Scope3/1, Product/1
  Demux/3 -> Terminator1/1
  Demux/2 -> Terminator/1
  Demux/1 -> To Workspace/1
  Gain1/1 -> Product/2
  k1/1 -> Gain1/1
  Gain/1 -> Product1/2
  k2/1 -> Gain/1
  Product/1 -> Reshape1/1
  Reshape1/1 -> Sum1/2
  Product1/1 -> Reshape2/1
  Transpose/1 -> Matrix Multiply/2
  Selector1/1 -> Mux/2
  Selector/1 -> Mux/1
  Selector2/1 -> Mux/3
  Reshape/1 -> Product1/1
  Sum1/1 -> Scope2/1, u/1
  Reshape2/1 -> Sum1/1
  Sum/1 -> Selector1/1, Selector/1, Selector2/1
  Transpose1/1 -> Sum/1
  Matrix Multiply/1 -> Transpose1/1, Sum/2
  A_BN_actual/1 -> Matrix Multiply/1, Scope1/1
  A_desired/1 -> Transpose/1

== system Main_simulation_gio/Slew Manouevre "quaternion" ==
  actual quaternion : Inport
  A_BN_desired : Inport  Port=2
  ω : Inport  Port=3
  A_B_N to quaternion : Subsystem
  Creation of Q_euler1 : Subsystem
  Demux : Demux
  Gain : Gain  Gain=-1
  Gain2 : Gain  Gain=-2
  Mux : Mux  Inputs=3
  Product : Product  Multiplication=Matrix(*)
  Product1 : Product
  Product2 : Product  Inputs=3
  Reshape : Reshape  OutputDimensionality=Column vector (2-D)
  Scope : Scope
  Scope1 : Scope
  Scope2 : Scope
  Sum : Sum  Inputs=|+|+|
  k1 : Constant  Value=0.5
  k2 : Constant  Value=1e-4
  M_c : Outport
  wires:
  actual quaternion/1 -> Product/2
  Creation of Q_euler1/1(Q_desired) -> Product/1
  A_BN_desired/1 -> A_B_N to quaternion/1(A_B_N from Euler)
  A_B_N to quaternion/1(q_euler) -> Creation of Q_euler1/1(q_desired)
  k1/1 -> Gain/1
  Gain/1 -> Product1/1
  ω/1 -> Scope/1, Product1/2
  [q_error] -> Product2/3
  Product1/1 -> Sum/1
  Product2/1 -> Sum/2
  Product/1 -> Scope1/1, Demux/1
  Demux/1 -> [qe1]
  Demux/4 -> [qe4]
  Demux/3 -> [qe3]
  Demux/2 -> [qe2]
  [qe1] -> Mux/1
  [qe2] -> Mux/2
  [qe3] -> Mux/3
  Mux/1 -> Reshape/1
  Reshape/1 -> Scope2/1, [q_error]
  k2/1 -> Product2/1
  [qe4] -> Gain2/1
  Gain2/1 -> Product2/2
  Sum/1 -> M_c/1

== system Main_simulation_gio/Subsystem1 ==
  b_b : Inport
  omega : Inport  Port=2
  K : Inport  Port=3
  Cross Product : matrix_library/Cross Product
      settings: SourceProductBaseCode=SL
  Cross Product1 : matrix_library/Cross Product
      settings: SourceProductBaseCode=SL
  Divide : Product  Inputs=/*
  Dot Product : DotProduct  InputSameDT=on  OutDataTypeStr=Inherit: Inherit via internal rule
  Gain : Gain  Gain=-1
  Product : Product
  M_c : Outport
  wires:
  b_b/1 -> Cross Product/1, Dot Product/2, Dot Product/1, Cross Product1/2
  omega/1 -> Cross Product/2
  Dot Product/1 -> Divide/1
  Cross Product/1 -> Divide/2
  Divide/1 -> Product/1
  Product/1 -> Cross Product1/1
  Cross Product1/1 -> M_c/1
  K/1 -> Gain/1
  Gain/1 -> Product/2

== system Main_simulation_gio/Sun Pointing 1 ==
  A_B_N from attitude determination : Inport
  S_N : Inport  Port=2
  A_B_N from Euler : Inport  Port=3
  Pointing error with DCM : Subsystem
  Pointing error with quaternions : Subsystem
  Difference between real and detected pointing error : Outport
  real pointing error : Outport  Port=2
  detected pointig error : Outport  Port=3
  A_BN_des : Outport  Port=4
  real error DCM : Outport  Port=5
  detected error DCM : Outport  Port=6
  wires:
  A_B_N from attitude determination/1 -> Pointing error with quaternions/1(A_B_N from attitude determination), Pointing error with DCM/3(A_B_N from attitude determination)
  S_N/1 -> Pointing error with quaternions/2(S_N), Pointing error with DCM/2(S_N)
  A_B_N from Euler/1 -> Pointing error with quaternions/3(A_B_N from Euler), Pointing error with DCM/1(A_B_N from Euler)
  Pointing error with DCM/1(Difference between real and detected pointing error) -> Difference between real and detected pointing error/1
  Pointing error with quaternions/2(detected pointing error) -> detected pointig error/1
  Pointing error with quaternions/1(real pointing error) -> real pointing error/1
  Pointing error with quaternions/3(q_euler) -> ?
  Pointing error with quaternions/4(q_desired) -> ?
  Pointing error with DCM/4(A_BN_des) -> A_BN_des/1
  Pointing error with DCM/2(real error DCM) -> real error DCM/1
  Pointing error with DCM/3(Detected error DCM) -> detected error DCM/1

== system Main_simulation_gio/Target Tracking ==
  A_BN_actual : Inport
  A_desired : Inport  Port=2
  w_measured : Inport  Port=3
  I_SC : Inport  Port=4
  Cross Product : matrix_library/Cross Product
      settings: SourceProductBaseCode=SL
  Demux : Demux  Outputs=3
  Gain : Gain  Gain=-1
  Gain1 : Gain  Gain=-1
  Matrix Multiply : Product  Multiplication=Matrix(*)
  Matrix Multiply1 : Product  Multiplication=Matrix(*)
  Mux : Mux  Inputs=3
  Product : Product
  Product1 : Product
  Reshape : Reshape  OutputDimensionality=Customize  OutputDimensions=[3,1]
  Reshape1 : Reshape  OutputDimensionality=Column vector (2-D)
  Reshape2 : Reshape  OutputDimensionality=Column vector (2-D)
  Scope{,1..4} (5 alike) : Scope
  Selector : Selector  NumberOfDimensions=2  InputPortWidth=3  IndexOptions=Index vector (dialog),Index vector (dialog)  Indices=2,1  OutputSizes=1,1
  Selector1 : Selector  NumberOfDimensions=2  InputPortWidth=3  IndexOptions=Index vector (dialog),Index vector (dialog)  Indices=3,1  OutputSizes=1,1
  Selector2 : Selector  NumberOfDimensions=2  InputPortWidth=3  IndexOptions=Index vector (dialog),Index vector (dialog)  Indices=3,2  OutputSizes=1,1
  Sum : Sum  Inputs=|+|-|
  Sum1 : Sum  Inputs=|+|+|+|
  Terminator : Terminator
  Terminator1 : Terminator
  To Workspace : ToWorkspace  VariableName=error  SaveFormat=Timeseries  SampleTime=-1
  To Workspace1 : ToWorkspace  VariableName=omega  SaveFormat=Timeseries  SampleTime=-1
  Transpose : Math  Operator=transpose  SaturateOnIntegerOverflow=on
  Transpose1 : Math  Operator=transpose  SaturateOnIntegerOverflow=on
  k1 : Constant  Value=9.99e-2
  k2 : Constant  Value=1.5e-3
  u : Outport
  wires:
  A_desired/1 -> Scope4/1, Transpose/1
  A_BN_actual/1 -> Scope1/1, Matrix Multiply/1
  Matrix Multiply/1 -> Sum/2, Transpose1/1
  Transpose1/1 -> Sum/1
  Sum/1 -> Selector2/1, Selector/1, Selector1/1
  Reshape2/1 -> Sum1/1
  Sum1/1 -> u/1, Scope2/1
  Reshape/1 -> Product1/1
  Selector2/1 -> Mux/3
  Selector/1 -> Mux/1
  Selector1/1 -> Mux/2
  Transpose/1 -> Matrix Multiply/2
  Product1/1 -> Reshape2/1
  Reshape1/1 -> Sum1/2
  Product/1 -> Reshape1/1
  k2/1 -> Gain/1
  Gain/1 -> Product1/2
  k1/1 -> Gain1/1
  Gain1/1 -> Product/2
  Demux/1 -> To Workspace/1
  Demux/2 -> Terminator/1
  Demux/3 -> Terminator1/1
  [I_mat] -> Matrix Multiply1/1
  w_measured/1 -> Matrix Multiply1/2, Cross Product/1, Product/1, Scope3/1, To Workspace1/1
  Cross Product/1 -> Sum1/3
  I_SC/1 -> [I_mat]
  Mux/1 -> Scope/1, Demux/1, Reshape/1
  Matrix Multiply1/1 -> Cross Product/2

== system Main_simulation_gio/Attitude determination/If Action Subsystem ==
  In1 : Inport
  Action Port : ActionPort  ActionPortLabel=if(u1 == u2)
  Out1 : Outport
  wires:
  In1/1 -> Out1/1

== system Main_simulation_gio/Attitude determination/If Action Subsystem1 ==
  In1 : Inport
  Action Port : ActionPort  ActionPortLabel=if(u1 == u2)
  Out1 : Outport
  wires:
  In1/1 -> Out1/1

== system Main_simulation_gio/Attitude determination/If Action Subsystem2 ==
  In1 : Inport
  Action Port : ActionPort  ActionPortLabel=if(u1 == u2)
  Out1 : Outport
  wires:
  In1/1 -> Out1/1

== system Main_simulation_gio/Attitude determination/If Action Subsystem3 ==
  In1 : Inport
  Action Port : ActionPort  ActionPortLabel=if(u1 == u2)
  Out1 : Outport
  wires:
  In1/1 -> Out1/1

== system Main_simulation_gio/Attitude determination/Subsystem ==
  b_sens : Inport
  b_N : Inport  Port=2
  Sun_sens : Inport  Port=3
  S_N : Inport  Port=4
  acc_magnetometre : Inport  Port=5
  acc_sun sensor : Inport  Port=6
  Add : Sum
  Add1 : Sum
  Divide : Product  Inputs=*/
  Divide1 : Product  Inputs=*/
  Matrix Multiply : Product  Multiplication=Matrix(*)
  Matrix Multiply1 : Product  Multiplication=Matrix(*)
  Normalize Vector : vrlib/Utilities/Normalize Vector  maxzero=0
  Normalize Vector1 : vrlib/Utilities/Normalize Vector  maxzero=0
  Product : Product
  Product1 : Product
  Transpose : Math  Operator=transpose  SaturateOnIntegerOverflow=on
  Transpose1 : Math  Operator=transpose  SaturateOnIntegerOverflow=on
  B : Outport
  wires:
  Transpose/1 -> Matrix Multiply1/2
  b_N/1 -> Normalize Vector1/1
  S_N/1 -> Transpose1/1
  Divide1/1 -> Product1/2
  Normalize Vector/1 -> Matrix Multiply1/1
  Add/1 -> B/1
  Divide/1 -> Product/2
  Product/1 -> Add/1
  b_sens/1 -> Normalize Vector/1
  Add1/1 -> Divide/2, Divide1/2
  [alpha2] -> Divide1/1
  [alpha1] -> Divide/1
  [alpha1] -> Add1/1
  Transpose1/1 -> Matrix Multiply/2
  acc_sun sensor/1 -> [alpha2]
  Matrix Multiply/1 -> Product1/1
  Matrix Multiply1/1 -> Product/1
  [alpha2] -> Add1/2
  acc_magnetometre/1 -> [alpha1]
  Normalize Vector1/1 -> Transpose/1
  Product1/1 -> Add/2
  Sun_sens/1 -> Matrix Multiply/1

== system Main_simulation_gio/Attitude determination/g to DCM ==
  In1 : Inport
  A_BN : Outport
  wires:
  In1/1 -> A_BN/1

== system Main_simulation_gio/Attitude determination/q to DCM ==
  In1 : Inport
  Add : Sum  Inputs=+-
  Add1 : Sum  Inputs=++-
  Constant : Constant  Value=[1 0 0; 0 1 0; 0 0 1]  VectorParams1D=off
  Demux : Demux
  Gain : Gain  Gain=2
  Gain1 : Gain  Gain=2
  Matrix Multiply : Product  Multiplication=Matrix(*)
  Matrix Multiply2 : Product  Multiplication=Matrix(*)
  Mux : Mux  Inputs=3
  Product : Product
  Product1 : Product
  Product2 : Product
  Reshape : Reshape  OutputDimensionality=Column vector (2-D)
  Reshape1 : Reshape  OutputDimensionality=Customize  OutputDimensions=[3,3]
  Scope : Scope
  Square : Math  Operator=square  SaturateOnIntegerOverflow=on
  Transpose : Math  Operator=transpose  SaturateOnIntegerOverflow=on
  Transpose1 : Math  Operator=transpose  SaturateOnIntegerOverflow=on
  Transpose2 : Math  Operator=transpose  SaturateOnIntegerOverflow=on
  orthonormalization step 1 : Subsystem
  q_cross : Subsystem
  A_BN : Outport
  wires:
  In1/1 -> Demux/1
  Demux/4 -> [q4]
  Demux/1 -> [q1]
  Demux/2 -> [q2]
  Demux/3 -> [q3]
  [q4] -> Square/1
  [q2] -> Mux/2
  [q3] -> Mux/3
  [q1] -> Mux/1
  Mux/1 -> Reshape/1
  Reshape/1 -> [q_vect]
  [q_vect] -> Matrix Multiply/2, Transpose/1
  Transpose/1 -> Matrix Multiply/1
  Matrix Multiply/1 -> Add/2
  Square/1 -> Add/1
  Constant/1 -> Reshape1/1
  Reshape1/1 -> Product1/2
  Product1/1 -> Add1/1
  Matrix Multiply2/1 -> Gain/1
  Gain/1 -> Add1/2
  Transpose1/1 -> Matrix Multiply2/2
  [q_vect] -> Transpose1/1, Matrix Multiply2/1
  Gain1/1 -> Add1/3
  Product/1 -> Gain1/1
  [q4] -> Product/2
  q_cross/1(q_cross) -> Product/1
  Add1/1 -> orthonormalization step 1/1(A*(t))
  [q_vect] -> q_cross/1(q_vect)
  Add/1 -> Product1/1
  Transpose2/1 -> Product2/2
  Product2/1 -> Scope/1
  orthonormalization step 1/1(A_BN*_filtered) -> A_BN/1, Product2/1, Transpose2/1

== system Main_simulation_gio/Enviroment/Gravity gradient ==
  I_SC : Inport
  A_BL : Inport  Port=2
  n : Inport  Port=3
  Constant : Constant  Value=3
  Constant1 : Constant  Value=[1 0 0]
  Demux : Demux  Outputs=9
  Demux1 : Demux  Outputs=3
  Matrix Multiply : Product  Multiplication=Matrix(*)
  Mux : Mux  Inputs=3
  Product{,1..9} (10 alike) : Product
  Reshape : Reshape  OutputDimensionality=Column vector (2-D)
  Reshape1 : Reshape  OutputDimensionality=Column vector (2-D)
  Reshape2 : Reshape  OutputDimensionality=Column vector (2-D)
  Scope : Scope  NumInputPorts=3
  Square : Math  Operator=square  SaturateOnIntegerOverflow=on
  Sum : Sum  Inputs=+-
  Sum1 : Sum  Inputs=+-
  Sum2 : Sum  Inputs=+-
  Terminator{,1..5} (6 alike) : Terminator
  T_GG : Outport
  wires:
  Demux/4 -> Terminator2/1
  Demux1/1 -> Product5/2, Product7/2
  Demux/2 -> Terminator/1
  Product6/1 -> Product9/1
  Sum/1 -> Product1/1
  Product1/1 -> Product6/1
  Demux/7 -> Terminator4/1
  Demux1/3 -> Product6/2, Product8/2
  Demux/1 -> Sum1/1
  Product5/1 -> Product8/1
  Demux/3 -> Terminator1/1
  I_SC/1 -> Reshape1/1
  Matrix Multiply/1 -> Demux1/1
  Demux/9 -> Sum2/2, Sum1/2, Sum/1
  Constant1/1 -> Reshape/1
  Sum1/1 -> Product2/1
  Sum2/1 -> Product3/1
  Product7/1 -> Scope/3, Mux/3
  Mux/1 -> Reshape2/1
  Demux/5 -> Sum/2, Sum2/1
  Demux/8 -> Terminator5/1
  A_BL/1 -> Matrix Multiply/1
  Product4/1 -> Product7/1
  Product8/1 -> Scope/2, Mux/2
  Demux/6 -> Terminator3/1
  Demux1/2 -> Product4/2, Product9/2
  Product2/1 -> Product5/1
  Product9/1 -> Scope/1, Mux/1
  Product3/1 -> Product4/1
  Reshape/1 -> Matrix Multiply/2
  Reshape1/1 -> Demux/1
  Reshape2/1 -> T_GG/1
  Square/1 -> Product/1
  Product/1 -> Product2/2, Product1/2, Product3/2
  Constant/1 -> Product/2
  n/1 -> Square/1

== system Main_simulation_gio/Enviroment/Magnetic field ==
  R : Inport
  A_BN : Inport  Port=2
  r_LVLH : Inport  Port=3
  Cross Product : matrix_library/Cross Product
      settings: SourceProductBaseCode=SL
  b_B : Subsystem
  parasitic torque : Subsystem
  T_B : Outport
  b_N : Outport  Port=2
  wires:
  parasitic torque/1(m_par) -> [m_par]
  b_B/1(b_B) -> [b_B]
  b_B/2(b_N) -> [b_N]
  [m_par] -> Cross Product/1
  [b_B] -> Cross Product/2
  [b_N] -> b_N/1
  A_BN/1 -> [A_BN]
  R/1 -> [R]
  r_LVLH/1 -> [r_LVLH]
  [A_BN] -> b_B/1(A_BN)
  [R] -> b_B/2(R)
  [r_LVLH] -> b_B/3(r_LVLH)
  Cross Product/1 -> T_B/1

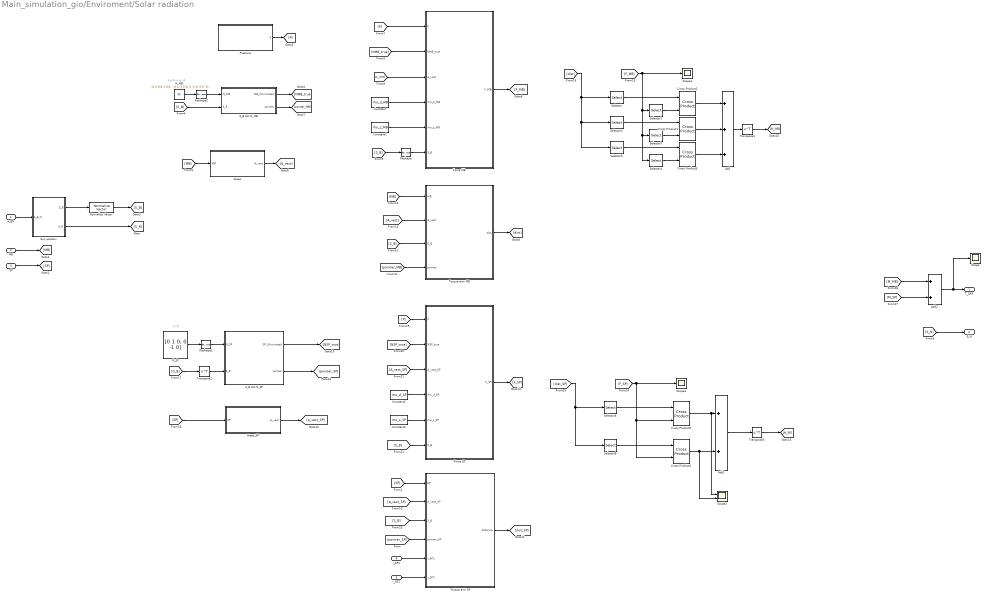
== system Main_simulation_gio/Enviroment/Solar radiation ==
  note: x,y,z,-x,-y,-z
  note: y,-y
  A_BN : Inport
  MB : Inport  Port=2
  SP : Inport  Port=3
  r_SP1 : Inport  Port=4
  r_SP2 : Inport  Port=5
  Add : Sum  Inputs=3
  Add1 : Sum
  Add2 : Sum
  Areas : Subsystem
  Areas_SP : Subsystem
  Constant : Constant  Value=rho_d_MB
  Constant1 : Constant  Value=rho_s_MB
  Constant2 : Constant  Value=rho_d_SP
  Constant3 : Constant  Value=rho_s_SP
  Cross Product{1..5} (5 alike) : matrix_library/Cross Product
      settings: SourceProductBaseCode=SL
  Force MB : Subsystem
  Force SP : Subsystem
  N_MB : Constant  Value=[1 0 0;0 1 0;0 0 1;-1 0 0; 0 -1 0; 0 0 -1]  VectorParams1D=off
  N_SP : Constant  Value=[0 1 0; 0 -1 0]  VectorParams1D=off
  Normalize Vector : vrlib/Utilities/Normalize Vector  maxzero=0
  Pressure : Subsystem
  Reshape : Reshape  OutputDimensionality=Column vector (2-D)
  Reshape1 : Reshape  OutputDimensionality=Customize  OutputDimensions=[2,3]
  Reshape2 : Reshape  OutputDimensionality=Customize  OutputDimensions=[6,3]
  S_B dot N_MB : Subsystem
  S_B dot N_SP : Subsystem
  Scope : Scope
  Scope1 : Scope
  Scope2 : Scope  NumInputPorts=2
  Scope3 : Scope
  Selector : Selector  NumberOfDimensions=2  InputPortWidth=3  IndexOptions=Index vector (dialog),Index vector (dialog)  Indices=1,[1 2 3]  OutputSizes=1,1
  Selector1 : Selector  NumberOfDimensions=2  InputPortWidth=3  IndexOptions=Index vector (dialog),Index vector (dialog)  Indices=1,[1 2 3]  OutputSizes=1,1
  Selector2 : Selector  NumberOfDimensions=2  InputPortWidth=3  IndexOptions=Index vector (dialog),Index vector (dialog)  Indices=2,[1 2 3]  OutputSizes=1,1
  Selector3 : Selector  NumberOfDimensions=2  InputPortWidth=3  IndexOptions=Index vector (dialog),Index vector (dialog)  Indices=2,[1 2 3]  OutputSizes=1,1
  Selector4 : Selector  NumberOfDimensions=2  InputPortWidth=3  IndexOptions=Index vector (dialog),Index vector (dialog)  Indices=3,[1 2 3]  OutputSizes=1,1
  Selector5 : Selector  NumberOfDimensions=2  InputPortWidth=3  IndexOptions=Index vector (dialog),Index vector (dialog)  Indices=3,[1 2 3]  OutputSizes=1,1
  Selector6 : Selector  NumberOfDimensions=2  InputPortWidth=3  IndexOptions=Index vector (dialog),Index vector (dialog)  Indices=1,[1 2 3]  OutputSizes=1,1
  Selector8 : Selector  NumberOfDimensions=2  InputPortWidth=3  IndexOptions=Index vector (dialog),Index vector (dialog)  Indices=2,[1 2 3]  OutputSizes=1,1
  Sun position : Subsystem
  Torque arm MB : Subsystem
  Torque arm SP : Subsystem
  Transpose1 : Math  Operator=transpose  SaturateOnIntegerOverflow=on
  Transpose2 : Math  Operator=transpose  SaturateOnIntegerOverflow=on
  Transpose3 : Math  Operator=transpose  SaturateOnIntegerOverflow=on
  T_SRP : Outport
  S_N : Outport  Port=2
  wires:
  A_BN/1 -> Sun position/1(A_B_N)
  Sun position/1(S_B) -> Normalize Vector/1
  Normalize Vector/1 -> [S_B]
  r_SP1/1 -> Torque arm SP/5(r_SP1)
  r_SP2/1 -> Torque arm SP/6(r_SP2)
  MB/1 -> [MB]
  SP/1 -> [SP]
  Sun position/2(S_N) -> [S_N]
  [S_N] -> S_N/1
  N_MB/1 -> Reshape2/1
  S_B dot N_MB/1(MB_illuminated) -> [NMB_true]
  [NMB_true] -> Force MB/2(NMB_true)
  [S_B] -> S_B dot N_MB/2(S_B)
  [MB] -> Areas/1(MB)
  Pressure/1(P) -> [P]
  Areas/1(A_vect) -> [A_vect]
  [P] -> Force MB/1(P)
  [A_vect] -> Force MB/3(A_vect)
  Constant/1 -> Force MB/4(rho_d_MB)
  Constant1/1 -> Force MB/5(rho_s_MB)
  [S_B] -> Reshape/1
  S_B dot N_MB/2(pointer) -> [pointer_MB]
  [pointer_MB] -> Torque arm MB/4(pointer)
  [S_B] -> Torque arm MB/3(S_B)
  [A_vect] -> Torque arm MB/2(A_vect)
  [MB] -> Torque arm MB/1(MB)
  Reshape/1 -> Force MB/6(S_B)
  Cross Product2/1 -> Add/1
  Selector/1 -> Cross Product2/1
  Selector1/1 -> Cross Product2/2
  Selector3/1 -> Cross Product1/2
  Selector2/1 -> Cross Product1/1
  [dist] -> Selector2/1, Selector5/1, Selector/1
  Cross Product1/1 -> Add/2
  Force MB/1(F_MB) -> [F_MB]
  [F_MB] -> Scope1/1, Selector4/1, Selector3/1, Selector1/1
  Cross Product3/1 -> Add/3
  Selector4/1 -> Cross Product3/2
  Selector5/1 -> Cross Product3/1
  Add/1 -> Transpose1/1
  Torque arm MB/1(dist) -> [dist]
  S_B dot N_SP/2(pointer) -> [pointer_SP]
  Areas_SP/1(A_vect) -> [A_vect_SP]
  [SP] -> Areas_SP/1(SP)
  Transpose2/1 -> S_B dot N_SP/2(S_B)
  [S_B] -> Transpose2/1
  S_B dot N_SP/1(SP_illuminated) -> [NSP_true]
  N_SP/1 -> Reshape1/1
  Reshape1/1 -> S_B dot N_SP/1(N_SP)
  Reshape2/1 -> S_B dot N_MB/1(N_MB)
  [P] -> Force SP/1(P)
  [NSP_true] -> Force SP/2(NSP_true)
  [A_vect_SP] -> Force SP/3(A_vect_SP)
  Constant2/1 -> Force SP/4(rho_d_SP)
  Constant3/1 -> Force SP/5(rho_s_SP)
  [S_B] -> Force SP/6(S_B)
  [pointer_SP] -> Torque arm SP/4(pointer_SP)
  [SP] -> Torque arm SP/1(SP)
  [A_vect_SP] -> Torque arm SP/2(A_vect_SP)
  [S_B] -> Torque arm SP/3(S_B)
  Torque arm SP/1(distance) -> [dist_SP]
  Force SP/1(F_SP) -> [F_SP]
  Transpose3/1 -> [M_SP]
  Add1/1 -> Transpose3/1
  Cross Product4/1 -> Scope2/2, Add1/2
  [dist_SP] -> Selector6/1, Selector8/1
  Selector8/1 -> Cross Product4/1
  [F_SP] -> Cross Product5/2, Cross Product4/2, Scope3/1
  Selector6/1 -> Cross Product5/1
  Cross Product5/1 -> Scope2/1, Add1/1
  Transpose1/1 -> [M_MB]
  [M_MB] -> Add2/1
  Add2/1 -> Scope/1, T_SRP/1
  [M_SP] -> Add2/2

== system Main_simulation_gio/Inertia matrix/Main body ==
  m_MB : Inport
  a_MB : Inport  Port=2
  b_MB : Inport  Port=3
  h_MB : Inport  Port=4
  Constant : Constant  Value=0
  Gain : Gain  Gain=1/12
  Gain1 : Gain  Gain=1/12
  Gain2 : Gain  Gain=1/12
  Product : Product
  Product1 : Product
  Product2 : Product
  Reshape : Reshape  OutputDimensionality=Customize  OutputDimensions=[3,3]
  Square : Math  Operator=square  SaturateOnIntegerOverflow=on
  Square1 : Math  Operator=square  SaturateOnIntegerOverflow=on
  Square2 : Math  Operator=square  SaturateOnIntegerOverflow=on
  Sum : Sum
  Sum1 : Sum
  Sum2 : Sum
  Vector Concatenate : Concatenate  NumInputs=9
  I_MB : Outport
  wires:
  Constant/1 -> Vector Concatenate/2, Vector Concatenate/3, Vector Concatenate/7, Vector Concatenate/8, Vector Concatenate/6, Vector Concatenate/4
  Square/1 -> Sum2/1, Sum1/1
  Square1/1 -> Sum2/2, Sum/1
  Square2/1 -> Sum/2, Sum1/2
  Product1/1 -> Gain1/1
  Gain/1 -> Vector Concatenate/1
  Product2/1 -> Gain2/1
  Sum1/1 -> Product1/2
  m_MB/1 -> Product/1, Product2/1, Product1/1
  Sum2/1 -> Product2/2
  a_MB/1 -> Square/1
  Vector Concatenate/1 -> Reshape/1
  Sum/1 -> Product/2
  b_MB/1 -> Square1/1
  Gain1/1 -> Vector Concatenate/5
  Product/1 -> Gain/1
  Gain2/1 -> Vector Concatenate/9
  Reshape/1 -> I_MB/1
  h_MB/1 -> Square2/1

== system Main_simulation_gio/Inertia matrix/Solar panel ==
  note: The inertia matrix for the solar panels is for two solar panels since they are the same and they are on opposite sides the distance vector between the centers of mass are one the opposite of the other and in the transport theorem the sign does not matter since I need only the norm and the d'*d that has + sign anyway
      | Still the mass and all characteristics are about one solar panel
  m_SP : Inport
  a_SP : Inport  Port=2
  b_SP : Inport  Port=3
  h_SP : Inport  Port=4
  Gain : Gain  Gain=1/12
  Gain1 : Gain  Gain=1/12
  Gain2 : Gain  Gain=1/12
  Gain3 : Gain  Gain=2
  Ground : Ground
  Product : Product
  Product1 : Product
  Product2 : Product
  Reshape : Reshape  OutputDimensionality=Customize  OutputDimensions=[3,3]
  Square : Math  Operator=square  SaturateOnIntegerOverflow=on
  Square1 : Math  Operator=square  SaturateOnIntegerOverflow=on
  Square2 : Math  Operator=square  SaturateOnIntegerOverflow=on
  Sum : Sum
  Sum1 : Sum
  Sum2 : Sum
  Vector Concatenate : Concatenate  NumInputs=9
  I_SP : Outport
  wires:
  Vector Concatenate/1 -> Reshape/1
  m_SP/1 -> Product/1, Product2/1, Product1/1
  Product/1 -> Gain/1
  Gain/1 -> Vector Concatenate/1
  Product1/1 -> Gain1/1
  Product2/1 -> Gain2/1
  Gain2/1 -> Vector Concatenate/9
  h_SP/1 -> Square/1
  a_SP/1 -> Square1/1
  b_SP/1 -> Square2/1
  Sum/1 -> Product/2
  Sum1/1 -> Product1/2
  Sum2/1 -> Product2/2
  Ground/1 -> Vector Concatenate/2, Vector Concatenate/3, Vector Concatenate/7, Vector Concatenate/8, Vector Concatenate/6, Vector Concatenate/4
  Gain1/1 -> Vector Concatenate/5
  Reshape/1 -> Gain3/1
  Gain3/1 -> I_SP/1
  Square1/1 -> Sum1/2, Sum2/1
  Square2/1 -> Sum/2, Sum2/2
  Square/1 -> Sum/1, Sum1/1
